simulink model "workingGT3nomasknwithcontrol"  (R2024a)
settings: Solver=ode15s  StartTime=0.0  StopTime=3600*48  RelTol=0.0001
model workspace (MAT data in the model file):
  TempGrad = 15
  Ti = 5
  roomarea1 = 20
libraries: fl_lib x2433, nesl_utility x241, SimscapeFluids_lib x137
(part 3 of 41)

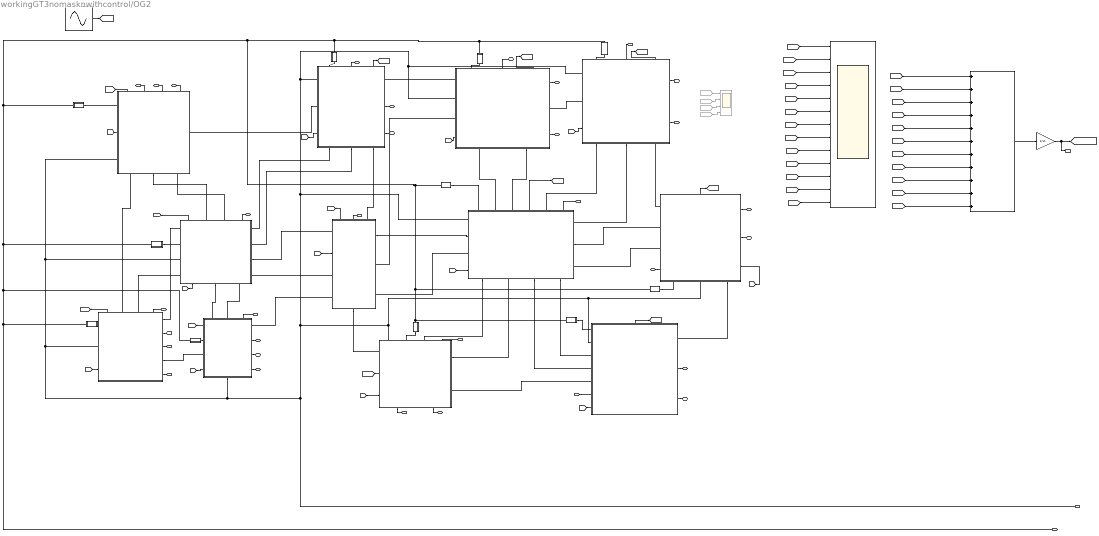
== system workingGT3nomasknwithcontrol/OG2 ==
  From : From  Commented=on  GotoTag=Troom1
  From1 : From  Commented=on  GotoTag=Troom2
  From2 : From  Commented=on  GotoTag=Troom3
  From3 : From  Commented=on  GotoTag=Troom4
  OG2 : Scope  NumInputPorts=13
  Pipe to 10 : Subsystem
  Pipe to 11 : Subsystem
  Pipe to 12 : Subsystem
  Pipe to 2 : Subsystem
  Pipe to 4 : Subsystem
  Pipe to 5 : Subsystem
  Pipe to 6 : Subsystem
  Pipe to 7 : Subsystem
  Pipe to 8 : Subsystem
  Pipe to 9a : Subsystem
  Raum1 : Subsystem
      settings: PortSchema="{\"entries\":[{\"content\":{\"sides\":[{\"content\":{\"connectorIds\":[\"LConn1\",\"LConn2\",\"LConn3\"]},\"type\":\"ConnectorPlacement.EquallySpacedRectSide\",\"uuid\":\"258852ae-79b4-4e90-ae22-4154c858ab0a\"},{\"content\":{\"connectorIds\":[\"RConn1\",\"In1\",\"RConn2\",\"RConn3\"],\"side\":\"RIGHT\"},\"type\":\"ConnectorPlacement.EquallySpacedRectSide\",\"uuid\":\"36706832-f330-42ce-9a32-f145cdee4912\"},{\"content\":{\"connectorIds\":[\"LConn4\",\"LConn5\",\"Out1\"],\"side\":\"TOP\"},\"type\":\"ConnectorPlacement.EquallySpacedRectSide\",\"uuid\":\"5cf2347a-3520-447e-9561-2d1c8313f3cf\"},{\"content\":{\"connectorIds\":[\"RConn4\"],\"side\":\"BOTTOM\"},\"type\":\"ConnectorPlacement.EquallySpacedRectSide\",\"uuid\":\"b1588268-8d41-4423-8f6e-2c28bf9b13dc\"}]},\"type\":\"ConnectorPlacement.EquallySpacedConnector\",\"uuid\":\"6bed35e7-1d7a-421b-a1f8-39267ed9017d\"}],\"packageUris\":[\"http://schema.mathworks.com/mf0/Connector/R2020b\"],\"version\":\"1.0\"}"
  Raum10 : Subsystem
      settings: PortSchema="{\"entries\":[{\"content\":{\"sides\":[{\"content\":{\"connectorIds\":[\"LConn1\",\"LConn2\",\"LConn3\",\"In1\"]},\"type\":\"ConnectorPlacement.EquallySpacedRectSide\",\"uuid\":\"258852ae-79b4-4e90-ae22-4154c858ab0a\"},{\"content\":{\"connectorIds\":[\"RConn1\",\"RConn2\",\"RConn3\"],\"side\":\"RIGHT\"},\"type\":\"ConnectorPlacement.EquallySpacedRectSide\",\"uuid\":\"36706832-f330-42ce-9a32-f145cdee4912\"},{\"content\":{\"connectorIds\":[\"LConn4\",\"LConn5\",\"Out1\"],\"side\":\"TOP\"},\"type\":\"ConnectorPlacement.EquallySpacedRectSide\",\"uuid\":\"5cf2347a-3520-447e-9561-2d1c8313f3cf\"},{\"content\":{\"connectorIds\":[\"RConn4\",\"RConn5\"],\"side\":\"BOTTOM\"},\"type\":\"ConnectorPlacement.EquallySpacedRectSide\",\"uuid\":\"b1588268-8d41-4423-8f6e-2c28bf9b13dc\"}]},\"type\":\"ConnectorPlacement.EquallySpacedConnector\",\"uuid\":\"6bed35e7-1d7a-421b-a1f8-39267ed9017d\"}],\"packageUris\":[\"http://schema.mathworks.com/mf0/Connector/R2020b\"],\"version\":\"1.0\"}"
  Raum11 : Subsystem
      settings: PortSchema="{\"entries\":[{\"content\":{\"sides\":[{\"content\":{\"connectorIds\":[\"LConn1\",\"LConn2\",\"In1\"]},\"type\":\"ConnectorPlacement.EquallySpacedRectSide\",\"uuid\":\"258852ae-79b4-4e90-ae22-4154c858ab0a\"},{\"content\":{\"connectorIds\":[\"RConn1\",\"RConn2\",\"RConn3\"],\"side\":\"RIGHT\"},\"type\":\"ConnectorPlacement.EquallySpacedRectSide\",\"uuid\":\"36706832-f330-42ce-9a32-f145cdee4912\"},{\"content\":{\"connectorIds\":[\"LConn3\",\"LConn4\",\"Out1\"],\"side\":\"TOP\"},\"type\":\"ConnectorPlacement.EquallySpacedRectSide\",\"uuid\":\"5cf2347a-3520-447e-9561-2d1c8313f3cf\"},{\"content\":{\"connectorIds\":[\"RConn4\",\"RConn5\",\"RConn6\"],\"side\":\"BOTTOM\"},\"type\":\"ConnectorPlacement.EquallySpacedRectSide\",\"uuid\":\"b1588268-8d41-4423-8f6e-2c28bf9b13dc\"}]},\"type\":\"ConnectorPlacement.EquallySpacedConnector\",\"uuid\":\"6bed35e7-1d7a-421b-a1f8-39267ed9017d\"}],\"packageUris\":[\"http://schema.mathworks.com/mf0/Connector/R2020b\"],\"version\":\"1.0\"}"
  Raum12 : Subsystem
      settings: PortSchema="{\"entries\":[{\"content\":{\"sides\":[{\"content\":{\"connectorIds\":[\"LConn1\",\"In1\",\"LConn2\"]},\"type\":\"ConnectorPlacement.EquallySpacedRectSide\",\"uuid\":\"258852ae-79b4-4e90-ae22-4154c858ab0a\"},{\"content\":{\"connectorIds\":[\"RConn1\"],\"side\":\"RIGHT\"},\"type\":\"ConnectorPlacement.EquallySpacedRectSide\",\"uuid\":\"36706832-f330-42ce-9a32-f145cdee4912\"},{\"content\":{\"connectorIds\":[\"Out1\",\"LConn3\",\"LConn4\",\"LConn5\"],\"side\":\"TOP\"},\"type\":\"ConnectorPlacement.EquallySpacedRectSide\",\"uuid\":\"5cf2347a-3520-447e-9561-2d1c8313f3cf\"},{\"content\":{\"connectorIds\":[\"RConn2\",\"RConn3\",\"RConn4\"],\"side\":\"BOTTOM\"},\"type\":\"ConnectorPlacement.EquallySpacedRectSide\",\"uuid\":\"b1588268-8d41-4423-8f6e-2c28bf9b13dc\"}]},\"type\":\"ConnectorPlacement.EquallySpacedConnector\",\"uuid\":\"6bed35e7-1d7a-421b-a1f8-39267ed9017d\"}],\"packageUris\":[\"http://schema.mathworks.com/mf0/Connector/R2020b\"],\"version\":\"1.0\"}"
  Raum2 : Subsystem
      settings: PortSchema="{\"entries\":[{\"content\":{\"sides\":[{\"content\":{\"connectorIds\":[\"LConn1\",\"LConn2\",\"LConn3\",\"LConn4\"]},\"type\":\"ConnectorPlacement.EquallySpacedRectSide\",\"uuid\":\"258852ae-79b4-4e90-ae22-4154c858ab0a\"},{\"content\":{\"connectorIds\":[\"RConn1\",\"RConn2\",\"RConn3\",\"RConn4\"],\"side\":\"RIGHT\"},\"type\":\"ConnectorPlacement.EquallySpacedRectSide\",\"uuid\":\"36706832-f330-42ce-9a32-f145cdee4912\"},{\"content\":{\"connectorIds\":[\"Out1\",\"LConn5\",\"LConn6\",\"LConn7\"],\"side\":\"TOP\"},\"type\":\"ConnectorPlacement.EquallySpacedRectSide\",\"uuid\":\"5cf2347a-3520-447e-9561-2d1c8313f3cf\"},{\"content\":{\"connectorIds\":[\"In1\",\"RConn5\",\"RConn6\"],\"side\":\"BOTTOM\"},\"type\":\"ConnectorPlacement.EquallySpacedRectSide\",\"uuid\":\"b1588268-8d41-4423-8f6e-2c28bf9b13dc\"}]},\"type\":\"ConnectorPlacement.EquallySpacedConnector\",\"uuid\":\"6bed35e7-1d7a-421b-a1f8-39267ed9017d\"}],\"packageUris\":[\"http://schema.mathworks.com/mf0/Connector/R2020b\"],\"version\":\"1.0\"}"
  Raum3 : Subsystem
      settings: PortSchema="{\"entries\":[{\"content\":{\"sides\":[{\"content\":{\"connectorIds\":[\"LConn1\",\"LConn2\",\"In1\"]},\"type\":\"ConnectorPlacement.EquallySpacedRectSide\",\"uuid\":\"258852ae-79b4-4e90-ae22-4154c858ab0a\"},{\"content\":{\"connectorIds\":[\"RConn1\",\"RConn2\",\"RConn3\",\"RConn4\",\"RConn5\"],\"side\":\"RIGHT\"},\"type\":\"ConnectorPlacement.EquallySpacedRectSide\",\"uuid\":\"36706832-f330-42ce-9a32-f145cdee4912\"},{\"content\":{\"connectorIds\":[\"Out1\",\"LConn3\",\"LConn4\",\"LConn5\"],\"side\":\"TOP\"},\"type\":\"ConnectorPlacement.EquallySpacedRectSide\",\"uuid\":\"5cf2347a-3520-447e-9561-2d1c8313f3cf\"},{\"content\":{\"side\":\"BOTTOM\"},\"type\":\"ConnectorPlacement.EquallySpacedRectSide\",\"uuid\":\"b1588268-8d41-4423-8f6e-2c28bf9b13dc\"}]},\"type\":\"ConnectorPlacement.EquallySpacedConnector\",\"uuid\":\"6bed35e7-1d7a-421b-a1f8-39267ed9017d\"}],\"packageUris\":[\"http://schema.mathworks.com/mf0/Connector/R2020b\"],\"version\":\"1.0\"}"
  Raum4 : Subsystem
      settings: PortSchema="{\"entries\":[{\"content\":{\"sides\":[{\"content\":{\"connectorIds\":[\"Out1\",\"LConn1\",\"LConn2\",\"In1\"]},\"type\":\"ConnectorPlacement.EquallySpacedRectSide\",\"uuid\":\"258852ae-79b4-4e90-ae22-4154c858ab0a\"},{\"content\":{\"connectorIds\":[\"RConn1\",\"RConn2\",\"RConn3\",\"RConn4\"],\"side\":\"RIGHT\"},\"type\":\"ConnectorPlacement.EquallySpacedRectSide\",\"uuid\":\"36706832-f330-42ce-9a32-f145cdee4912\"},{\"content\":{\"connectorIds\":[\"LConn3\",\"LConn4\",\"LConn5\"],\"side\":\"TOP\"},\"type\":\"ConnectorPlacement.EquallySpacedRectSide\",\"uuid\":\"5cf2347a-3520-447e-9561-2d1c8313f3cf\"},{\"content\":{\"connectorIds\":[\"RConn5\"],\"side\":\"BOTTOM\"},\"type\":\"ConnectorPlacement.EquallySpacedRectSide\",\"uuid\":\"b1588268-8d41-4423-8f6e-2c28bf9b13dc\"}]},\"type\":\"ConnectorPlacement.EquallySpacedConnector\",\"uuid\":\"6bed35e7-1d7a-421b-a1f8-39267ed9017d\"}],\"packageUris\":[\"http://schema.mathworks.com/mf0/Connector/R2020b\"],\"version\":\"1.0\"}"
  Raum5 : Subsystem
      settings: PortSchema="{\"entries\":[{\"content\":{\"sides\":[{\"content\":{\"connectorIds\":[\"LConn1\",\"LConn2\",\"LConn3\",\"LConn4\"]},\"type\":\"ConnectorPlacement.EquallySpacedRectSide\",\"uuid\":\"258852ae-79b4-4e90-ae22-4154c858ab0a\"},{\"content\":{\"connectorIds\":[\"RConn1\",\"RConn2\",\"In1\"],\"side\":\"RIGHT\"},\"type\":\"ConnectorPlacement.EquallySpacedRectSide\",\"uuid\":\"36706832-f330-42ce-9a32-f145cdee4912\"},{\"content\":{\"connectorIds\":[\"Out1\"],\"side\":\"TOP\"},\"type\":\"ConnectorPlacement.EquallySpacedRectSide\",\"uuid\":\"5cf2347a-3520-447e-9561-2d1c8313f3cf\"},{\"content\":{\"connectorIds\":[\"RConn3\",\"RConn4\",\"RConn5\"],\"side\":\"BOTTOM\"},\"type\":\"ConnectorPlacement.EquallySpacedRectSide\",\"uuid\":\"b1588268-8d41-4423-8f6e-2c28bf9b13dc\"}]},\"type\":\"ConnectorPlacement.EquallySpacedConnector\",\"uuid\":\"6bed35e7-1d7a-421b-a1f8-39267ed9017d\"}],\"packageUris\":[\"http://schema.mathworks.com/mf0/Connector/R2020b\"],\"version\":\"1.0\"}"
  Raum6 : Subsystem
      settings: PortSchema="{\"entries\":[{\"content\":{\"sides\":[{\"content\":{\"connectorIds\":[\"LConn1\",\"LConn2\",\"LConn3\",\"LConn4\",\"LConn5\",\"LConn6\",\"In1\"]},\"type\":\"ConnectorPlacement.EquallySpacedRectSide\",\"uuid\":\"258852ae-79b4-4e90-ae22-4154c858ab0a\"},{\"content\":{\"connectorIds\":[\"RConn1\",\"RConn2\",\"RConn3\"],\"side\":\"RIGHT\"},\"type\":\"ConnectorPlacement.EquallySpacedRectSide\",\"uuid\":\"36706832-f330-42ce-9a32-f145cdee4912\"},{\"content\":{\"connectorIds\":[\"Out1\"],\"side\":\"TOP\"},\"type\":\"ConnectorPlacement.EquallySpacedRectSide\",\"uuid\":\"5cf2347a-3520-447e-9561-2d1c8313f3cf\"},{\"content\":{\"side\":\"BOTTOM\"},\"type\":\"ConnectorPlacement.EquallySpacedRectSide\",\"uuid\":\"b1588268-8d41-4423-8f6e-2c28bf9b13dc\"}]},\"type\":\"ConnectorPlacement.EquallySpacedConnector\",\"uuid\":\"6bed35e7-1d7a-421b-a1f8-39267ed9017d\"}],\"packageUris\":[\"http://schema.mathworks.com/mf0/Connector/R2020b\"],\"version\":\"1.0\"}"
  Raum7 : Subsystem
      settings: PortSchema="{\"entries\":[{\"content\":{\"sides\":[{\"content\":{\"connectorIds\":[\"LConn1\",\"LConn2\",\"LConn3\",\"In1\"]},\"type\":\"ConnectorPlacement.EquallySpacedRectSide\",\"uuid\":\"258852ae-79b4-4e90-ae22-4154c858ab0a\"},{\"content\":{\"connectorIds\":[\"RConn1\",\"RConn2\",\"RConn3\"],\"side\":\"RIGHT\"},\"type\":\"ConnectorPlacement.EquallySpacedRectSide\",\"uuid\":\"36706832-f330-42ce-9a32-f145cdee4912\"},{\"content\":{\"connectorIds\":[\"LConn4\",\"LConn5\",\"LConn6\",\"Out1\",\"LConn7\",\"LConn8\"],\"side\":\"TOP\"},\"type\":\"ConnectorPlacement.EquallySpacedRectSide\",\"uuid\":\"5cf2347a-3520-447e-9561-2d1c8313f3cf\"},{\"content\":{\"connectorIds\":[\"RConn4\",\"RConn5\",\"RConn6\",\"RConn7\"],\"side\":\"BOTTOM\"},\"type\":\"ConnectorPlacement.EquallySpacedRectSide\",\"uuid\":\"b1588268-8d41-4423-8f6e-2c28bf9b13dc\"}]},\"type\":\"ConnectorPlacement.EquallySpacedConnector\",\"uuid\":\"6bed35e7-1d7a-421b-a1f8-39267ed9017d\"}],\"packageUris\":[\"http://schema.mathworks.com/mf0/Connector/R2020b\"],\"version\":\"1.0\"}"
  Raum8 : Subsystem
      settings: PortSchema="{\"entries\":[{\"content\":{\"sides\":[{\"content\":{\"connectorIds\":[\"LConn1\",\"Out1\",\"In1\"]},\"type\":\"ConnectorPlacement.EquallySpacedRectSide\",\"uuid\":\"258852ae-79b4-4e90-ae22-4154c858ab0a\"},{\"content\":{\"connectorIds\":[\"RConn1\",\"RConn2\"],\"side\":\"RIGHT\"},\"type\":\"ConnectorPlacement.EquallySpacedRectSide\",\"uuid\":\"36706832-f330-42ce-9a32-f145cdee4912\"},{\"content\":{\"connectorIds\":[\"LConn2\",\"LConn3\",\"LConn4\",\"LConn5\"],\"side\":\"TOP\"},\"type\":\"ConnectorPlacement.EquallySpacedRectSide\",\"uuid\":\"5cf2347a-3520-447e-9561-2d1c8313f3cf\"},{\"content\":{\"connectorIds\":[\"RConn3\",\"RConn4\"],\"side\":\"BOTTOM\"},\"type\":\"ConnectorPlacement.EquallySpacedRectSide\",\"uuid\":\"b1588268-8d41-4423-8f6e-2c28bf9b13dc\"}]},\"type\":\"ConnectorPlacement.EquallySpacedConnector\",\"uuid\":\"6bed35e7-1d7a-421b-a1f8-39267ed9017d\"}],\"packageUris\":[\"http://schema.mathworks.com/mf0/Connector/R2020b\"],\"version\":\"1.0\"}"
  Raum9 : Subsystem
      settings: PortSchema="{\"entries\":[{\"content\":{\"sides\":[{\"content\":{\"connectorIds\":[\"LConn1\",\"LConn2\",\"In1\"]},\"type\":\"ConnectorPlacement.EquallySpacedRectSide\",\"uuid\":\"258852ae-79b4-4e90-ae22-4154c858ab0a\"},{\"content\":{\"connectorIds\":[\"RConn1\",\"RConn2\"],\"side\":\"RIGHT\"},\"type\":\"ConnectorPlacement.EquallySpacedRectSide\",\"uuid\":\"36706832-f330-42ce-9a32-f145cdee4912\"},{\"content\":{\"connectorIds\":[\"LConn3\",\"LConn4\",\"Out1\"],\"side\":\"TOP\"},\"type\":\"ConnectorPlacement.EquallySpacedRectSide\",\"uuid\":\"5cf2347a-3520-447e-9561-2d1c8313f3cf\"},{\"content\":{\"connectorIds\":[\"RConn3\",\"RConn4\",\"RConn5\"],\"side\":\"BOTTOM\"},\"type\":\"ConnectorPlacement.EquallySpacedRectSide\",\"uuid\":\"b1588268-8d41-4423-8f6e-2c28bf9b13dc\"}]},\"type\":\"ConnectorPlacement.EquallySpacedConnector\",\"uuid\":\"6bed35e7-1d7a-421b-a1f8-39267ed9017d\"}],\"packageUris\":[\"http://schema.mathworks.com/mf0/Connector/R2020b\"],\"version\":\"1.0\"}"
  RaumTemperaturverlauf : Scope  Commented=on  NumInputPorts=4
  Sum of Elements : Sum  Inputs=+++++++++++
  Tatm12 : Sin  Amplitude=7  Bias=5  Frequency=2*pi/(24*3600)  SampleTime=0
  TavgOG2 : Gain  Gain=1/11
  pipe to 3 : Subsystem
  hot water in : PMIOPort  Side=Left
  Hot Water Out1 : PMIOPort  Port=2  Side=Right
  Y-1 : PMIOPort  Port=3  Side=Right
  Y-3 : PMIOPort  Port=4  Side=Right
  Y-4 : PMIOPort  Port=5  Side=Right
  Y-5 : PMIOPort  Port=6  Side=Right
  Y-6 : PMIOPort  Port=7  Side=Right
  Y-8 : PMIOPort  Port=8  Side=Right
  Y-7 : PMIOPort  Port=9  Side=Right
  Y-9 : PMIOPort  Port=10  Side=Right
  Y-10 : PMIOPort  Port=11  Side=Right
  Y-11 : PMIOPort  Port=12  Side=Right
  Y-12 : PMIOPort  Port=13  Side=Right
  Y-13 : PMIOPort  Port=14  Side=Right
  Y-14 : PMIOPort  Port=15  Side=Right
  Y-15 : PMIOPort  Port=16  Side=Right
  Y-16 : PMIOPort  Port=17  Side=Right
  Y-17 : PMIOPort  Port=18  Side=Right
  Y-18 : PMIOPort  Port=19  Side=Right
  Y-19 : PMIOPort  Port=20  Side=Right
  Y-20 : PMIOPort  Port=21  Side=Right
  Y-21 : PMIOPort  Port=22  Side=Right
  Y-6 Flur12OG2 : PMIOPort  Port=23  Side=Right
  Y-Flur11OG2 : PMIOPort  Port=24  Side=Right
  Y-Flur10OG2 : PMIOPort  Port=25  Side=Right
  Y-Flur9OG2 : PMIOPort  Port=26  Side=Right
  Y-Flur8OG2 : PMIOPort  Port=27  Side=Right
  Y-Flur7OG2 : PMIOPort  Port=28  Side=Right
  Y-Flur6OG2 : PMIOPort  Port=29  Side=Right
  Y-Flur5OG2 : PMIOPort  Port=30  Side=Right
  Y-Flur4OG2 : PMIOPort  Port=31  Side=Right
  Y-Flur3OG2 : PMIOPort  Port=32  Side=Right
  Y-Flur2OG2 : PMIOPort  Port=33  Side=Right
  Y-Flur1OG2 : PMIOPort  Port=34  Side=Right
  Outport : Outport
  wires:
  Raum9/1(Troom) -> [Traum9]
  [Traum4] -> OG2/4
  [Traum10] -> OG2/10
  [Tatm] -> Raum11/1(Tatm)
  Raum6/1(Troom) -> [Traum6]
  [Traum5] -> OG2/5
  [Traum7] -> OG2/7
  [Tatm] -> Raum9/1(Tatm)
  Raum7/1(Troom) -> [Traum7]
  [Traum9] -> OG2/9
  [Tatm] -> Raum7/1(Tatm)
  From/1 -> RaumTemperaturverlauf/1
  [Traum12] -> OG2/12
  Raum11/1(Troom) -> [Troom11]
  [Traum6] -> OG2/6
  [Tatm] -> Raum2/1(Tatm)
  From2/1 -> RaumTemperaturverlauf/3
  Raum2/1(Troom) -> [Traum2]
  From3/1 -> RaumTemperaturverlauf/4
  [Tatm] -> Raum10/1(Tatm)
  [Tatm] -> Raum1/1(Tatm)
  [Tatm] -> Raum5/1(Tatm)
  [Tatm] -> Raum3/1(Tatm)
  [Traum1] -> OG2/1
  [Tatm] -> Raum4/1(Tatm)
  From1/1 -> RaumTemperaturverlauf/2
  [Traum2] -> OG2/2
  Raum3/1(Troom) -> [Traum3]
  Raum10/1(Troom) -> [Traum10]
  Raum1/1(Troom) -> [Traum1]
  [Tatm] -> Raum6/1(Tatm)
  [Traum3] -> OG2/3
  [Tatm] -> Raum8/1(Tatm)
  Raum4/1(Troom) -> [Traum4]
  Raum5/1(Troom) -> [Traum5]
  [Traum8] -> OG2/8
  [Troom11] -> OG2/11
  Raum8/1(Troom) -> [Traum8]
  Raum12/1(Troom) -> [Traum12]
  [Tatm] -> Raum12/1(Tatm)
  Tatm12/1 -> [Tatm]
  [TavgOG2] -> OG2/13
  TavgOG2/1 -> Outport/1, [TavgOG2]
  [Traum9] -> Sum of Elements/8
  [Traum6] -> Sum of Elements/5
  Sum of Elements/1 -> TavgOG2/1
  [Traum4] -> Sum of Elements/3
  [Traum5] -> Sum of Elements/4
  [Traum8] -> Sum of Elements/7
  [Traum7] -> Sum of Elements/6
  [Traum3] -> Sum of Elements/2
  [Traum2] -> Sum of Elements/1
  [Traum10] -> Sum of Elements/9
  [Troom11] -> Sum of Elements/10
  [Traum12] -> Sum of Elements/11
  connections:
  Raum6/LConn5 -- Raum8/RConn2
  Raum3/LConn2 -- Raum2/LConn3 -- Raum12/LConn2 -- Raum4/RConn5 -- Hot Water Out1/RConn1 -- Raum5/RConn4 -- Raum6/LConn2 -- Raum8/LConn2 -- Raum11/LConn1 -- Raum9/LConn1 -- Raum10/LConn2 -- Raum7/LConn1
  Raum5/RConn5 -- Raum6/RConn1
  Raum7/RConn6 -- Raum6/LConn4
  Pipe to 6/RConn1 -- Raum6/LConn1
  Raum11/RConn2 -- Y-3/RConn1
  Raum1/RConn2 -- Raum2/RConn4
  Pipe to 12/RConn1 -- Raum12/LConn1
  Pipe to 7/RConn1 -- Raum7/LConn4
  Raum11/LConn2 -- Raum12/RConn1
  Pipe to 4/LConn1 -- Pipe to 2/LConn1 -- Pipe to 11/LConn1 -- Pipe to 10/LConn1 -- Pipe to 9a/LConn1 -- Pipe to 7/LConn1 -- Pipe to 6/LConn1 -- Pipe to 8/LConn1 -- Pipe to 5/LConn1 -- Pipe to 12/LConn1 -- hot water in/RConn1 -- pipe to 3/LConn1
  Raum3/LConn4 -- Raum2/LConn4
  Raum4/LConn4 -- Raum2/RConn6
  Raum10/RConn3 -- Y-9/RConn1
  Raum11/RConn6 -- Raum1/LConn4
  Raum9/LConn3 -- Pipe to 9a/RConn1
  Raum5/LConn1 -- Raum9/RConn5
  Pipe to 4/RConn1 -- Raum4/LConn1
  Raum6/RConn2 -- Y-16/RConn1
  Raum4/RConn4 -- Y-17/RConn1
  Raum3/RConn5 -- Y-18/RConn1
  Raum7/RConn7 -- Raum6/LConn3
  Pipe to 8/RConn1 -- Raum8/LConn3
  Pipe to 11/RConn1 -- Raum11/LConn3
  Raum9/RConn4 -- Raum7/RConn1
  Raum10/LConn1 -- Raum11/RConn1
  Raum8/RConn3 -- Y-20/RConn1
  Raum2/LConn6 -- Raum12/RConn4
  Raum7/LConn3 -- Raum1/LConn3
  Pipe to 10/RConn1 -- Raum10/LConn4
  Raum10/RConn1 -- Y-1/RConn1
  Raum12/LConn5 -- Y-7/RConn1
  pipe to 3/RConn1 -- Raum3/LConn1
  Raum11/RConn3 -- Y-8/RConn1
  Raum1/RConn4 -- Raum8/LConn1
  Raum9/LConn2 -- Raum10/RConn2
  Raum5/LConn3 -- Raum7/RConn3
  Raum9/RConn1 -- Y-6/RConn1
  Raum2/RConn5 -- Raum4/LConn3
  Raum7/RConn4 -- Raum8/LConn4
  Raum3/LConn3 -- Raum12/RConn2
  Raum10/LConn3 -- Raum1/LConn2
  Pipe to 2/RConn1 -- Raum2/LConn2
  Raum12/RConn3 -- Raum2/LConn5
  Raum10/RConn5 -- Raum7/LConn6
  Raum7/RConn2 -- Raum5/LConn2
  Raum11/RConn4 -- Raum2/RConn1
  Raum3/RConn1 -- Raum2/LConn1
  Raum9/RConn3 -- Raum7/LConn7
  Raum3/RConn4 -- Raum4/LConn2
  Pipe to 5/RConn1 -- Raum5/RConn3
  Raum1/RConn3 -- Raum4/RConn1
  Raum1/LConn1 -- Raum7/LConn2
  Raum11/RConn5 -- Raum2/RConn2
  Raum8/RConn1 -- Raum7/RConn5
  Raum7/LConn5 -- Raum10/RConn4
  Raum2/RConn3 -- Raum1/RConn1
  Raum4/RConn3 -- Y-15/RConn1
  Raum5/RConn1 -- Y-10/RConn1
  Raum9/RConn2 -- Y-4/RConn1
  Raum5/RConn2 -- Y-11/RConn1
  Raum8/RConn4 -- Y-21/RConn1
  Raum12/LConn3 -- Y-5/RConn1
  Raum12/LConn4 -- Y-6 Flur12OG2/RConn1
  Raum3/RConn3 -- Y-14/RConn1
  Raum3/RConn2 -- Y-12/RConn1
  Raum4/RConn2 -- Y-13/RConn1
  Raum6/RConn3 -- Y-19/RConn1
  Raum11/LConn4 -- Y-Flur11OG2/RConn1
  Raum10/LConn5 -- Y-Flur10OG2/RConn1
  Raum9/LConn4 -- Y-Flur9OG2/RConn1
  Y-Flur5OG2/RConn1 -- Raum5/LConn4
  Raum7/LConn8 -- Y-Flur7OG2/RConn1
  Y-Flur6OG2/RConn1 -- Raum6/LConn6
  Y-Flur8OG2/RConn1 -- Raum8/LConn5
  Raum1/LConn5 -- Y-Flur1OG2/RConn1
  Y-Flur4OG2/RConn1 -- Raum4/LConn5
  Raum3/LConn5 -- Y-Flur3OG2/RConn1
  Raum2/LConn7 -- Y-Flur2OG2/RConn1

== system workingGT3nomasknwithcontrol/Pump//Velocity ==
  Centrifugal Pump (TL) : SimscapeFluids_lib/Thermal Liquid/Pumps & Motors/Centrifugal Pump (TL)  pump_parameterization=fluids.thermal_liquid.pumps_motors.enum.CentrifugalPumpParameterization.Table1D  capacity_ref_nominal=45 lpm  head_ref_nominal=40 m  power_ref_nominal=0.85 kW  head_ref_max=60 m  capacity_ref_max=80 lpm  omega_ref_analytic=1770 rpm  flow_rate_1D_TLU=[16.67, 30, 40, 53.33, 66.67, 83.33] lpm  head_1D_TLU=[50, 47.5, 45, 40, 35, 25] m  power_1D_TLU=[.6, .75, .85, .93, .98, .99] kW  omega_ref_1D=3500 rpm  rho_ref_1D=998.21 kg/m^3  omega_threshold_factor=1e-2  flow_rate_2D_TLU=[16.67, 23.33, 30, 40, 53.33, 60] lpm  omega_2D_TLU=[2450, 2800, 3150, 3500] rpm  head_2D_TLU=[25, 32.7, 42.5, 50; 24, 31.7, 41, 49; 22.7, 30.5, 39, 47.5; 20, 28, 36, 45; 15.7, 24, 32, 40; 12.5, 21, 29.5, 37.5] m  power_2D_TLU=[.28, .38, .5, .6; .31, .41, .55, .68; .33, .44, .6, .75; .36, .48, .65, .83; .38, .53, .72, .93; .39, .55, .75, .97] kW  rho_ref_2D=998.21 kg/m^3  diameter_ratio=1  mech_orientation=fluids.thermal_liquid.pumps_motors.enum.CentrifugalPumpMechOrientation.Positive  area=0.01 m^2  operation_check=simscape.enum.assert.action.none
      settings: InternalSimscapePortConfiguration="{\"Bottom\":[],\"Left\":[{\"id\":\"A\",\"label\":\"A\",\"type\":\"foundation.thermal_liquid.thermal_liquid\"},{\"id\":\"B\",\"label\":\"B\",\"type\":\"foundation.thermal_liquid.thermal_liquid\"}],\"Right\":[{\"id\":\"R\",\"label\":\"R\",\"type\":\"foundation.mechanical.rotational.rotational\"},{\"id\":\"C\",\"label\":\"C\",\"type\":\"foundation.mechanical.rotational.rotational\"}],\"Top\":[]}"
  Constant : Constant  Value=100
  Ideal Angular Velocity Source : fl_lib/Mechanical/Mechanical Sources/Ideal Angular Velocity Source
  Mechanical Rotational Reference : fl_lib/Mechanical/Rotational Elements/Mechanical Rotational Reference
  Simulink-PS Converter1 : nesl_utility/Simulink-PS Converter  PhysicalDomain=network_engine_domain  SubClassName=ps_input  LeftPortType=input  RightPortType=output  PseudoPeriodic=off  Frequencies=[]  NoiseDistribution=none  NoiseParameters=[]  Unit=1  AffineConversion=off  FilteringAndDerivatives=provide  SimscapeFilterOrder=1  InputFilterTimeConstant=0.001  UdotUserProvided=0
  OUT : PMIOPort  Side=Left
  IN : PMIOPort  Port=2  Side=Right
  wires:
  Constant/1 -> Simulink-PS Converter1/1
  connections:
  Ideal Angular Velocity Source/RConn2 -- Centrifugal Pump (TL)/RConn2 -- Mechanical Rotational Reference/LConn1
  IN/RConn1 -- Centrifugal Pump (TL)/LConn1
  Centrifugal Pump (TL)/LConn2 -- OUT/RConn1
  Ideal Angular Velocity Source/LConn1 -- Centrifugal Pump (TL)/RConn1
  Simulink-PS Converter1/RConn1 -- Ideal Angular Velocity Source/RConn1

== system workingGT3nomasknwithcontrol/Subsystem ==
  Heat Input : Inport
  Constant : Constant  Value=-1
  Constant2 : Constant  Value=-273
  Controlled Heat Flow Rate Source : fl_lib/Thermal/Thermal Sources/Controlled Heat Flow Rate Source
  Controller Relay : Relay  OnSwitchValue=-316  OffSwitchValue=-318  OffOutputValue=0.008
  PS-Simulink Converter : nesl_utility/PS-Simulink Converter  PhysicalDomain=network_engine_domain  SubClassName=ps_output  LeftPortType=input  RightPortType=output  PseudoPeriodic=off  Frequencies=[]  VectorFormat=inherit  Unit=inherit  AffineConversion=off
  Product : Product
  Product1 : Product
  Simulink-PS Converter : nesl_utility/Simulink-PS Converter  PhysicalDomain=network_engine_domain  SubClassName=ps_input  LeftPortType=input  RightPortType=output  PseudoPeriodic=off  Frequencies=[]  NoiseDistribution=none  NoiseParameters=[]  Unit=1  AffineConversion=off  FilteringAndDerivatives=provide  SimscapeFilterOrder=1  InputFilterTimeConstant=0.001  UdotUserProvided=0
  Sum : Sum  Inputs=|++
  Thermal Reference : fl_lib/Thermal/Thermal Elements/Thermal Reference
  Heat supply to tank : PMIOPort  Side=Left
  hot water temp : PMIOPort  Port=2  Side=Left
  Hot Water Temp : Outport
  wires:
  Product/1 -> Controller Relay/1
  Constant/1 -> Product/2
  Product1/1 -> Simulink-PS Converter/1
  Heat Input/1 -> Product1/1
  PS-Simulink Converter/1 -> Product/1, Sum/1
  Constant2/1 -> Sum/2
  Controller Relay/1 -> Product1/2
  Sum/1 -> Hot Water Temp/1
  connections:
  Simulink-PS Converter/RConn1 -- Controlled Heat Flow Rate Source/RConn1
  Thermal Reference/LConn1 -- Controlled Heat Flow Rate Source/RConn2
  Controlled Heat Flow Rate Source/LConn1 -- Heat supply to tank/RConn1
  hot water temp/RConn1 -- PS-Simulink Converter/LConn1

== system workingGT3nomasknwithcontrol/Ctrl 1/Controller 11 ==
  In1 : Inport
  In2 : Inport  Port=2
  Constant : Constant  Value=0.095
  Manual Switch : ManualSwitch
  Relay1 : Relay  OnSwitchValue=.5  OffSwitchValue=-.5  OnOutputValue=.095  OffOutputValue=0.002
  Simulink-PS Converter : nesl_utility/Simulink-PS Converter  PhysicalDomain=network_engine_domain  SubClassName=ps_input  LeftPortType=input  RightPortType=output  PseudoPeriodic=off  Frequencies=[]  NoiseDistribution=none  NoiseParameters=[]  Unit=1  AffineConversion=off  FilteringAndDerivatives=provide  SimscapeFilterOrder=1  InputFilterTimeConstant=0.001  UdotUserProvided=0
  Sum : Sum  Inputs=|+-
  output : PMIOPort  Side=Right
  wires:
  In2/1 -> Sum/2
  Constant/1 -> Manual Switch/2
  In1/1 -> Sum/1
  Sum/1 -> Relay1/1
  Manual Switch/1 -> Simulink-PS Converter/1
  Relay1/1 -> Manual Switch/1
  connections:
  Simulink-PS Converter/RConn1 -- output/RConn1

== system workingGT3nomasknwithcontrol/Ctrl 12/Controller 11 ==
  In1 : Inport
  In2 : Inport  Port=2
  Constant : Constant  Value=0.095
  Manual Switch : ManualSwitch
  Relay1 : Relay  OnSwitchValue=.5  OffSwitchValue=-.5  OnOutputValue=.095  OffOutputValue=0.002
  Simulink-PS Converter : nesl_utility/Simulink-PS Converter  PhysicalDomain=network_engine_domain  SubClassName=ps_input  LeftPortType=input  RightPortType=output  PseudoPeriodic=off  Frequencies=[]  NoiseDistribution=none  NoiseParameters=[]  Unit=1  AffineConversion=off  FilteringAndDerivatives=provide  SimscapeFilterOrder=1  InputFilterTimeConstant=0.001  UdotUserProvided=0
  Sum : Sum  Inputs=|+-
  output : PMIOPort  Side=Right
  wires:
  Sum/1 -> Relay1/1
  In1/1 -> Sum/1
  Constant/1 -> Manual Switch/2
  In2/1 -> Sum/2
  Manual Switch/1 -> Simulink-PS Converter/1
  Relay1/1 -> Manual Switch/1
  connections:
  Simulink-PS Converter/RConn1 -- output/RConn1

== system workingGT3nomasknwithcontrol/Ctrl 2/Controller 11 ==
  In1 : Inport
  In2 : Inport  Port=2
  Constant : Constant  Value=0.095
  Manual Switch : ManualSwitch
  Relay1 : Relay  OnSwitchValue=.5  OffSwitchValue=-.5  OnOutputValue=.095  OffOutputValue=0.002
  Simulink-PS Converter : nesl_utility/Simulink-PS Converter  PhysicalDomain=network_engine_domain  SubClassName=ps_input  LeftPortType=input  RightPortType=output  PseudoPeriodic=off  Frequencies=[]  NoiseDistribution=none  NoiseParameters=[]  Unit=1  AffineConversion=off  FilteringAndDerivatives=provide  SimscapeFilterOrder=1  InputFilterTimeConstant=0.001  UdotUserProvided=0
  Sum : Sum  Inputs=|+-
  output : PMIOPort  Side=Right
  wires:
  Sum/1 -> Relay1/1
  In1/1 -> Sum/1
  Constant/1 -> Manual Switch/2
  In2/1 -> Sum/2
  Relay1/1 -> Manual Switch/1
  Manual Switch/1 -> Simulink-PS Converter/1
  connections:
  Simulink-PS Converter/RConn1 -- output/RConn1

== system workingGT3nomasknwithcontrol/EG/Pipe to 10 ==
  Flow Rate Sensor (TL)1 : fl_lib/Thermal Liquid/Sensors/Flow Rate Sensor (TL)  mass_flow_measure=false  volumetric_flow_measure=true  energy_flow_measure=false
      settings: InternalSimscapePortConfiguration="{\"Bottom\":[],\"Left\":[{\"id\":\"A\",\"label\":\"A\",\"type\":\"foundation.thermal_liquid.thermal_liquid\"}],\"Right\":[{\"id\":\"B\",\"label\":\"B\",\"type\":\"foundation.thermal_liquid.thermal_liquid\"},{\"id\":\"V\",\"label\":\"V\",\"type\":\"output\"}],\"Top\":[]}"
  PS-Simulink Converter1 : nesl_utility/PS-Simulink Converter  PhysicalDomain=network_engine_domain  SubClassName=ps_output  LeftPortType=input  RightPortType=output  PseudoPeriodic=off  Frequencies=[]  VectorFormat=inherit  Unit=inherit  AffineConversion=off
  Perfect Insulator3 : fl_lib/Thermal/Thermal Elements/Perfect Insulator  T_specify=off  T_priority=None  T=293.15 K  T_nominal_specify=off  T_nominal_value=1  T_nominal_unit=K
  Pipe (TL)3 : fl_lib/Thermal Liquid/Elements/Pipe (TL)  length=5.88 m  area=0.01 m^2  Dh=0.1128 m  length_add=1 m  roughness=15e-6 m  Re_lam=2000  Re_tur=4000  shape_factor=64  Nu_lam=3.66  dynamic_compressibility=true  inertia=false  p0=0.101325 MPa  T0=293.15 K  mdot0=0 kg/s
  Hot Water In1 : PMIOPort  Side=Right
  Conn2 : PMIOPort  Port=2  Side=Left
  wires:
  PS-Simulink Converter1/1 -> [FR2]
  connections:
  Perfect Insulator3/LConn1 -- Pipe (TL)3/LConn2
  PS-Simulink Converter1/LConn1 -- Flow Rate Sensor (TL)1/RConn2
  Flow Rate Sensor (TL)1/LConn1 -- Pipe (TL)3/RConn1
  Flow Rate Sensor (TL)1/RConn1 -- Hot Water In1/RConn1
  Conn2/RConn1 -- Pipe (TL)3/LConn1

== system workingGT3nomasknwithcontrol/EG/Pipe to 11 ==
  Flow Rate Sensor (TL)1 : fl_lib/Thermal Liquid/Sensors/Flow Rate Sensor (TL)  mass_flow_measure=false  volumetric_flow_measure=true  energy_flow_measure=false
      settings: InternalSimscapePortConfiguration="{\"Bottom\":[],\"Left\":[{\"id\":\"A\",\"label\":\"A\",\"type\":\"foundation.thermal_liquid.thermal_liquid\"}],\"Right\":[{\"id\":\"B\",\"label\":\"B\",\"type\":\"foundation.thermal_liquid.thermal_liquid\"},{\"id\":\"V\",\"label\":\"V\",\"type\":\"output\"}],\"Top\":[]}"
  PS-Simulink Converter1 : nesl_utility/PS-Simulink Converter  PhysicalDomain=network_engine_domain  SubClassName=ps_output  LeftPortType=input  RightPortType=output  PseudoPeriodic=off  Frequencies=[]  VectorFormat=inherit  Unit=inherit  AffineConversion=off
  Perfect Insulator3 : fl_lib/Thermal/Thermal Elements/Perfect Insulator  T_specify=off  T_priority=None  T=293.15 K  T_nominal_specify=off  T_nominal_value=1  T_nominal_unit=K
  Pipe (TL)3 : fl_lib/Thermal Liquid/Elements/Pipe (TL)  length=5.32 m  area=0.01 m^2  Dh=0.1128 m  length_add=1 m  roughness=15e-6 m  Re_lam=2000  Re_tur=4000  shape_factor=64  Nu_lam=3.66  dynamic_compressibility=true  inertia=false  p0=0.101325 MPa  T0=293.15 K  mdot0=0 kg/s
  Hot Water In1 : PMIOPort  Side=Right
  Conn2 : PMIOPort  Port=2  Side=Left
  wires:
  PS-Simulink Converter1/1 -> [FR2]
  connections:
  Conn2/RConn1 -- Pipe (TL)3/LConn1
  Flow Rate Sensor (TL)1/RConn1 -- Hot Water In1/RConn1
  Flow Rate Sensor (TL)1/LConn1 -- Pipe (TL)3/RConn1
  PS-Simulink Converter1/LConn1 -- Flow Rate Sensor (TL)1/RConn2
  Perfect Insulator3/LConn1 -- Pipe (TL)3/LConn2

== system workingGT3nomasknwithcontrol/EG/Pipe to 12 ==
  Flow Rate Sensor (TL)1 : fl_lib/Thermal Liquid/Sensors/Flow Rate Sensor (TL)  mass_flow_measure=false  volumetric_flow_measure=true  energy_flow_measure=false
      settings: InternalSimscapePortConfiguration="{\"Bottom\":[],\"Left\":[{\"id\":\"A\",\"label\":\"A\",\"type\":\"foundation.thermal_liquid.thermal_liquid\"}],\"Right\":[{\"id\":\"B\",\"label\":\"B\",\"type\":\"foundation.thermal_liquid.thermal_liquid\"},{\"id\":\"V\",\"label\":\"V\",\"type\":\"output\"}],\"Top\":[]}"
  PS-Simulink Converter1 : nesl_utility/PS-Simulink Converter  PhysicalDomain=network_engine_domain  SubClassName=ps_output  LeftPortType=input  RightPortType=output  PseudoPeriodic=off  Frequencies=[]  VectorFormat=inherit  Unit=inherit  AffineConversion=off
  Perfect Insulator3 : fl_lib/Thermal/Thermal Elements/Perfect Insulator  T_specify=off  T_priority=None  T=293.15 K  T_nominal_specify=off  T_nominal_value=1  T_nominal_unit=K
  Pipe (TL)3 : fl_lib/Thermal Liquid/Elements/Pipe (TL)  length=7.7 m  area=0.01 m^2  Dh=0.1128 m  length_add=1 m  roughness=15e-6 m  Re_lam=2000  Re_tur=4000  shape_factor=64  Nu_lam=3.66  dynamic_compressibility=true  inertia=false  p0=0.101325 MPa  T0=293.15 K  mdot0=0 kg/s
  Conn1 : PMIOPort  Side=Right
  Conn2 : PMIOPort  Port=2  Side=Left
  wires:
  PS-Simulink Converter1/1 -> [FR2]
  connections:
  Perfect Insulator3/LConn1 -- Pipe (TL)3/LConn2
  PS-Simulink Converter1/LConn1 -- Flow Rate Sensor (TL)1/RConn2
  Flow Rate Sensor (TL)1/LConn1 -- Pipe (TL)3/RConn1
  Flow Rate Sensor (TL)1/RConn1 -- Conn1/RConn1
  Conn2/RConn1 -- Pipe (TL)3/LConn1

== system workingGT3nomasknwithcontrol/EG/Pipe to 2 ==
  Flow Rate Sensor (TL)3 : fl_lib/Thermal Liquid/Sensors/Flow Rate Sensor (TL)  mass_flow_measure=false  volumetric_flow_measure=true  energy_flow_measure=false
      settings: InternalSimscapePortConfiguration="{\"Bottom\":[],\"Left\":[{\"id\":\"A\",\"label\":\"A\",\"type\":\"foundation.thermal_liquid.thermal_liquid\"}],\"Right\":[{\"id\":\"B\",\"label\":\"B\",\"type\":\"foundation.thermal_liquid.thermal_liquid\"},{\"id\":\"V\",\"label\":\"V\",\"type\":\"output\"}],\"Top\":[]}"
  PS-Simulink Converter3 : nesl_utility/PS-Simulink Converter  PhysicalDomain=network_engine_domain  SubClassName=ps_output  LeftPortType=input  RightPortType=output  PseudoPeriodic=off  Frequencies=[]  VectorFormat=inherit  Unit=inherit  AffineConversion=off
  Perfect Insulator1 : fl_lib/Thermal/Thermal Elements/Perfect Insulator  T_specify=off  T_priority=None  T=293.15 K  T_nominal_specify=off  T_nominal_value=1  T_nominal_unit=K
  Pipe (TL)1 : fl_lib/Thermal Liquid/Elements/Pipe (TL)  length=2.38 m  area=0.01 m^2  Dh=0.1128 m  length_add=1 m  roughness=15e-6 m  Re_lam=2000  Re_tur=4000  shape_factor=64  Nu_lam=3.66  dynamic_compressibility=true  inertia=false  p0=0.101325 MPa  T0=293.15 K  mdot0=0 kg/s
  Conn1 : PMIOPort  Side=Left
  Conn2 : PMIOPort  Port=2  Side=Right
  wires:
  PS-Simulink Converter3/1 -> [FR4]
  connections:
  Flow Rate Sensor (TL)3/RConn1 -- Conn2/RConn1
  Flow Rate Sensor (TL)3/LConn1 -- Pipe (TL)1/RConn1
  Flow Rate Sensor (TL)3/RConn2 -- PS-Simulink Converter3/LConn1
  Perfect Insulator1/LConn1 -- Pipe (TL)1/LConn2
  Conn1/RConn1 -- Pipe (TL)1/LConn1

== system workingGT3nomasknwithcontrol/EG/Pipe to 4 ==
  Flow Rate Sensor (TL)2 : fl_lib/Thermal Liquid/Sensors/Flow Rate Sensor (TL)  mass_flow_measure=false  volumetric_flow_measure=true  energy_flow_measure=false
      settings: InternalSimscapePortConfiguration="{\"Bottom\":[],\"Left\":[{\"id\":\"A\",\"label\":\"A\",\"type\":\"foundation.thermal_liquid.thermal_liquid\"}],\"Right\":[{\"id\":\"B\",\"label\":\"B\",\"type\":\"foundation.thermal_liquid.thermal_liquid\"},{\"id\":\"V\",\"label\":\"V\",\"type\":\"output\"}],\"Top\":[]}"
  PS-Simulink Converter2 : nesl_utility/PS-Simulink Converter  PhysicalDomain=network_engine_domain  SubClassName=ps_output  LeftPortType=input  RightPortType=output  PseudoPeriodic=off  Frequencies=[]  VectorFormat=inherit  Unit=inherit  AffineConversion=off
  Perfect Insulator2 : fl_lib/Thermal/Thermal Elements/Perfect Insulator  T_specify=off  T_priority=None  T=293.15 K  T_nominal_specify=off  T_nominal_value=1  T_nominal_unit=K
  Pipe (TL)2 : fl_lib/Thermal Liquid/Elements/Pipe (TL)  length=7.38 m  area=0.01 m^2  Dh=0.1128 m  length_add=1 m  roughness=15e-6 m  Re_lam=2000  Re_tur=4000  shape_factor=64  Nu_lam=3.66  dynamic_compressibility=true  inertia=false  p0=0.101325 MPa  T0=293.15 K  mdot0=0 kg/s
  Conn1 : PMIOPort  Side=Left
  Conn2 : PMIOPort  Port=2  Side=Right
  wires:
  PS-Simulink Converter2/1 -> [FR3]
  connections:
  Perfect Insulator2/LConn1 -- Pipe (TL)2/LConn2
  PS-Simulink Converter2/LConn1 -- Flow Rate Sensor (TL)2/RConn2
  Pipe (TL)2/LConn1 -- Conn1/RConn1
  Flow Rate Sensor (TL)2/RConn1 -- Conn2/RConn1
  Flow Rate Sensor (TL)2/LConn1 -- Pipe (TL)2/RConn1

== system workingGT3nomasknwithcontrol/EG/Pipe to 5 ==
  Flow Rate Sensor (TL)1 : fl_lib/Thermal Liquid/Sensors/Flow Rate Sensor (TL)  mass_flow_measure=false  volumetric_flow_measure=true  energy_flow_measure=false
      settings: InternalSimscapePortConfiguration="{\"Bottom\":[],\"Left\":[{\"id\":\"A\",\"label\":\"A\",\"type\":\"foundation.thermal_liquid.thermal_liquid\"}],\"Right\":[{\"id\":\"B\",\"label\":\"B\",\"type\":\"foundation.thermal_liquid.thermal_liquid\"},{\"id\":\"V\",\"label\":\"V\",\"type\":\"output\"}],\"Top\":[]}"
  PS-Simulink Converter1 : nesl_utility/PS-Simulink Converter  PhysicalDomain=network_engine_domain  SubClassName=ps_output  LeftPortType=input  RightPortType=output  PseudoPeriodic=off  Frequencies=[]  VectorFormat=inherit  Unit=inherit  AffineConversion=off
  Perfect Insulator3 : fl_lib/Thermal/Thermal Elements/Perfect Insulator  T_specify=off  T_priority=None  T=293.15 K  T_nominal_specify=off  T_nominal_value=1  T_nominal_unit=K
  Pipe (TL)3 : fl_lib/Thermal Liquid/Elements/Pipe (TL)  length=12.42 m  area=0.01 m^2  Dh=0.1128 m  length_add=1 m  roughness=15e-6 m  Re_lam=2000  Re_tur=4000  shape_factor=64  Nu_lam=3.66  dynamic_compressibility=true  inertia=false  p0=0.101325 MPa  T0=293.15 K  mdot0=0 kg/s
  Hot Water In1 : PMIOPort  Side=Right
  Conn2 : PMIOPort  Port=2  Side=Left
  wires:
  PS-Simulink Converter1/1 -> [FR2]
  connections:
  Perfect Insulator3/LConn1 -- Pipe (TL)3/LConn2
  PS-Simulink Converter1/LConn1 -- Flow Rate Sensor (TL)1/RConn2
  Flow Rate Sensor (TL)1/LConn1 -- Pipe (TL)3/RConn1
  Flow Rate Sensor (TL)1/RConn1 -- Hot Water In1/RConn1
  Conn2/RConn1 -- Pipe (TL)3/LConn1

== system workingGT3nomasknwithcontrol/EG/Pipe to 6 ==
  Flow Rate Sensor (TL)1 : fl_lib/Thermal Liquid/Sensors/Flow Rate Sensor (TL)  mass_flow_measure=false  volumetric_flow_measure=true  energy_flow_measure=false
      settings: InternalSimscapePortConfiguration="{\"Bottom\":[],\"Left\":[{\"id\":\"A\",\"label\":\"A\",\"type\":\"foundation.thermal_liquid.thermal_liquid\"}],\"Right\":[{\"id\":\"B\",\"label\":\"B\",\"type\":\"foundation.thermal_liquid.thermal_liquid\"},{\"id\":\"V\",\"label\":\"V\",\"type\":\"output\"}],\"Top\":[]}"
  PS-Simulink Converter1 : nesl_utility/PS-Simulink Converter  PhysicalDomain=network_engine_domain  SubClassName=ps_output  LeftPortType=input  RightPortType=output  PseudoPeriodic=off  Frequencies=[]  VectorFormat=inherit  Unit=inherit  AffineConversion=off
  Perfect Insulator3 : fl_lib/Thermal/Thermal Elements/Perfect Insulator  T_specify=off  T_priority=None  T=293.15 K  T_nominal_specify=off  T_nominal_value=1  T_nominal_unit=K
  Pipe (TL)3 : fl_lib/Thermal Liquid/Elements/Pipe (TL)  length=9.34 m  area=0.01 m^2  Dh=0.1128 m  length_add=1 m  roughness=15e-6 m  Re_lam=2000  Re_tur=4000  shape_factor=64  Nu_lam=3.66  dynamic_compressibility=true  inertia=false  p0=0.101325 MPa  T0=293.15 K  mdot0=0 kg/s
  Hot Water In1 : PMIOPort  Side=Right
  Conn2 : PMIOPort  Port=2  Side=Left
  wires:
  PS-Simulink Converter1/1 -> [FR2]
  connections:
  Conn2/RConn1 -- Pipe (TL)3/LConn1
  Flow Rate Sensor (TL)1/RConn1 -- Hot Water In1/RConn1
  Flow Rate Sensor (TL)1/LConn1 -- Pipe (TL)3/RConn1
  PS-Simulink Converter1/LConn1 -- Flow Rate Sensor (TL)1/RConn2
  Perfect Insulator3/LConn1 -- Pipe (TL)3/LConn2

== system workingGT3nomasknwithcontrol/EG/Pipe to 7 ==
  Flow Rate Sensor (TL)1 : fl_lib/Thermal Liquid/Sensors/Flow Rate Sensor (TL)  mass_flow_measure=false  volumetric_flow_measure=true  energy_flow_measure=false
      settings: InternalSimscapePortConfiguration="{\"Bottom\":[],\"Left\":[{\"id\":\"A\",\"label\":\"A\",\"type\":\"foundation.thermal_liquid.thermal_liquid\"}],\"Right\":[{\"id\":\"B\",\"label\":\"B\",\"type\":\"foundation.thermal_liquid.thermal_liquid\"},{\"id\":\"V\",\"label\":\"V\",\"type\":\"output\"}],\"Top\":[]}"
  PS-Simulink Converter1 : nesl_utility/PS-Simulink Converter  PhysicalDomain=network_engine_domain  SubClassName=ps_output  LeftPortType=input  RightPortType=output  PseudoPeriodic=off  Frequencies=[]  VectorFormat=inherit  Unit=inherit  AffineConversion=off
  Perfect Insulator3 : fl_lib/Thermal/Thermal Elements/Perfect Insulator  T_specify=off  T_priority=None  T=293.15 K  T_nominal_specify=off  T_nominal_value=1  T_nominal_unit=K
  Pipe (TL)3 : fl_lib/Thermal Liquid/Elements/Pipe (TL)  length=3.5 m  area=0.01 m^2  Dh=0.1128 m  length_add=1 m  roughness=15e-6 m  Re_lam=2000  Re_tur=4000  shape_factor=64  Nu_lam=3.66  dynamic_compressibility=true  inertia=false  p0=0.101325 MPa  T0=293.15 K  mdot0=0 kg/s
  Hot Water In1 : PMIOPort  Side=Right
  Conn2 : PMIOPort  Port=2  Side=Left
  wires:
  PS-Simulink Converter1/1 -> [FR2]
  connections:
  Perfect Insulator3/LConn1 -- Pipe (TL)3/LConn2
  PS-Simulink Converter1/LConn1 -- Flow Rate Sensor (TL)1/RConn2
  Flow Rate Sensor (TL)1/LConn1 -- Pipe (TL)3/RConn1
  Flow Rate Sensor (TL)1/RConn1 -- Hot Water In1/RConn1
  Conn2/RConn1 -- Pipe (TL)3/LConn1

== system workingGT3nomasknwithcontrol/EG/Pipe to 8 ==
  Flow Rate Sensor (TL)1 : fl_lib/Thermal Liquid/Sensors/Flow Rate Sensor (TL)  mass_flow_measure=false  volumetric_flow_measure=true  energy_flow_measure=false
      settings: InternalSimscapePortConfiguration="{\"Bottom\":[],\"Left\":[{\"id\":\"A\",\"label\":\"A\",\"type\":\"foundation.thermal_liquid.thermal_liquid\"}],\"Right\":[{\"id\":\"B\",\"label\":\"B\",\"type\":\"foundation.thermal_liquid.thermal_liquid\"},{\"id\":\"V\",\"label\":\"V\",\"type\":\"output\"}],\"Top\":[]}"
  PS-Simulink Converter1 : nesl_utility/PS-Simulink Converter  PhysicalDomain=network_engine_domain  SubClassName=ps_output  LeftPortType=input  RightPortType=output  PseudoPeriodic=off  Frequencies=[]  VectorFormat=inherit  Unit=inherit  AffineConversion=off
  Perfect Insulator3 : fl_lib/Thermal/Thermal Elements/Perfect Insulator  T_specify=off  T_priority=None  T=293.15 K  T_nominal_specify=off  T_nominal_value=1  T_nominal_unit=K
  Pipe (TL)3 : fl_lib/Thermal Liquid/Elements/Pipe (TL)  length=10.04 m  area=0.01 m^2  Dh=0.1128 m  length_add=1 m  roughness=15e-6 m  Re_lam=2000  Re_tur=4000  shape_factor=64  Nu_lam=3.66  dynamic_compressibility=true  inertia=false  p0=0.101325 MPa  T0=293.15 K  mdot0=0 kg/s
  Hot Water In1 : PMIOPort  Side=Right
  Conn2 : PMIOPort  Port=2  Side=Left
  wires:
  PS-Simulink Converter1/1 -> [FR2]
  connections:
  Perfect Insulator3/LConn1 -- Pipe (TL)3/LConn2
  PS-Simulink Converter1/LConn1 -- Flow Rate Sensor (TL)1/RConn2
  Flow Rate Sensor (TL)1/LConn1 -- Pipe (TL)3/RConn1
  Flow Rate Sensor (TL)1/RConn1 -- Hot Water In1/RConn1
  Conn2/RConn1 -- Pipe (TL)3/LConn1

== system workingGT3nomasknwithcontrol/EG/Pipe to 9a ==
  Flow Rate Sensor (TL)1 : fl_lib/Thermal Liquid/Sensors/Flow Rate Sensor (TL)  mass_flow_measure=false  volumetric_flow_measure=true  energy_flow_measure=false
      settings: InternalSimscapePortConfiguration="{\"Bottom\":[],\"Left\":[{\"id\":\"A\",\"label\":\"A\",\"type\":\"foundation.thermal_liquid.thermal_liquid\"}],\"Right\":[{\"id\":\"B\",\"label\":\"B\",\"type\":\"foundation.thermal_liquid.thermal_liquid\"},{\"id\":\"V\",\"label\":\"V\",\"type\":\"output\"}],\"Top\":[]}"
  PS-Simulink Converter1 : nesl_utility/PS-Simulink Converter  PhysicalDomain=network_engine_domain  SubClassName=ps_output  LeftPortType=input  RightPortType=output  PseudoPeriodic=off  Frequencies=[]  VectorFormat=inherit  Unit=inherit  AffineConversion=off
  Perfect Insulator3 : fl_lib/Thermal/Thermal Elements/Perfect Insulator  T_specify=off  T_priority=None  T=293.15 K  T_nominal_specify=off  T_nominal_value=1  T_nominal_unit=K
  Pipe (TL)3 : fl_lib/Thermal Liquid/Elements/Pipe (TL)  length=10.14 m  area=0.01 m^2  Dh=0.1128 m  length_add=1 m  roughness=15e-6 m  Re_lam=2000  Re_tur=4000  shape_factor=64  Nu_lam=3.66  dynamic_compressibility=true  inertia=false  p0=0.101325 MPa  T0=293.15 K  mdot0=0 kg/s
  Hot Water In1 : PMIOPort  Side=Right
  Conn2 : PMIOPort  Port=2  Side=Left
  wires:
  PS-Simulink Converter1/1 -> [FR2]
  connections:
  Conn2/RConn1 -- Pipe (TL)3/LConn1
  Flow Rate Sensor (TL)1/RConn1 -- Hot Water In1/RConn1
  Flow Rate Sensor (TL)1/LConn1 -- Pipe (TL)3/RConn1
  PS-Simulink Converter1/LConn1 -- Flow Rate Sensor (TL)1/RConn2
  Perfect Insulator3/LConn1 -- Pipe (TL)3/LConn2
